simulink model "Microgrid_W"  (R2020a)
settings: Solver=ode15s  StartTime=0  StopTime=1440*1  MaxStep=1  RelTol=1e-3
libraries: simulink x4214, powerlib x685, simulink_extras x28, Microgrid_Library x18, powerlib_meascontrol x12
(part 39 of 48)

== system Microgrid_W/House 5 W1/Light 5/D5 ==
  Clock : Clock
  Constant : Constant
  Constant1 : Constant  Value=0
  Gain : Gain  Gain=t
  Interval Test : simulink/Logic and Bit Operations/Interval Test  IntervalClosedRight=on  uplimit=K_L4_Off_1+86400*4  IntervalClosedLeft=on  lowlimit=K_L4_On_1+86400*4  OutDataTypeStr=boolean
  Switch : Switch  Criteria=u2 > Threshold  Threshold=0.5
  Out1 : Outport  VectorParamsAs1DForOutWhenUnconnected=off
  wires:
  Clock/1 -> Gain/1
  Gain/1 -> Interval Test/1
  Constant/1 -> Switch/1
  Constant1/1 -> Switch/3
  Switch/1 -> Out1/1
  Interval Test/1 -> Switch/2

== system Microgrid_W/House 5 W1/Light 5/D6 ==
  Clock : Clock
  Constant : Constant
  Constant1 : Constant  Value=0
  Gain : Gain  Gain=t
  Interval Test : simulink/Logic and Bit Operations/Interval Test  IntervalClosedRight=on  uplimit=K_L4_Off_1+86400*5  IntervalClosedLeft=on  lowlimit=K_L4_On_1+86400*5  OutDataTypeStr=boolean
  Switch : Switch  Criteria=u2 > Threshold  Threshold=0.5
  Out1 : Outport  VectorParamsAs1DForOutWhenUnconnected=off
  wires:
  Clock/1 -> Gain/1
  Interval Test/1 -> Switch/2
  Switch/1 -> Out1/1
  Constant1/1 -> Switch/3
  Constant/1 -> Switch/1
  Gain/1 -> Interval Test/1

== system Microgrid_W/House 5 W1/Light 5/D7 ==
  Clock : Clock
  Constant : Constant
  Constant1 : Constant  Value=0
  Gain : Gain  Gain=t
  Interval Test : simulink/Logic and Bit Operations/Interval Test  IntervalClosedRight=on  uplimit=K_L4_Off_1+86400*6  IntervalClosedLeft=on  lowlimit=K_L4_On_1+86400*6  OutDataTypeStr=boolean
  Switch : Switch  Criteria=u2 > Threshold  Threshold=0.5
  Out1 : Outport  VectorParamsAs1DForOutWhenUnconnected=off
  wires:
  Clock/1 -> Gain/1
  Gain/1 -> Interval Test/1
  Constant/1 -> Switch/1
  Constant1/1 -> Switch/3
  Switch/1 -> Out1/1
  Interval Test/1 -> Switch/2

== system Microgrid_W/House 5 W1/Light 6/D1 ==
  Add : Sum
  Clock : Clock
  Constant : Constant
  Constant1 : Constant  Value=0
  Gain : Gain  Gain=t
  Interval Test : simulink/Logic and Bit Operations/Interval Test  IntervalClosedRight=on  uplimit=K_L5_Off_1  IntervalClosedLeft=on  lowlimit=K_L5_On_1  OutDataTypeStr=boolean
  Interval Test1 : simulink/Logic and Bit Operations/Interval Test  IntervalClosedRight=on  uplimit=K_L5_Off_2  IntervalClosedLeft=on  lowlimit=K_L5_On_2  OutDataTypeStr=boolean
  Switch : Switch  Criteria=u2 > Threshold  Threshold=0.5
  Switch1 : Switch  Criteria=u2 > Threshold  Threshold=0.5
  Out1 : Outport  VectorParamsAs1DForOutWhenUnconnected=off
  wires:
  Clock/1 -> Gain/1
  Interval Test/1 -> Switch/2
  Switch/1 -> Add/1
  Interval Test1/1 -> Switch1/2
  Add/1 -> Out1/1
  Constant1/1 -> Switch/3, Switch1/3
  Constant/1 -> Switch/1, Switch1/1
  Switch1/1 -> Add/2
  Gain/1 -> Interval Test1/1, Interval Test/1

== system Microgrid_W/House 5 W1/Light 6/D2 ==
  Add : Sum
  Clock : Clock
  Constant : Constant
  Constant1 : Constant  Value=0
  Gain : Gain  Gain=t
  Interval Test : simulink/Logic and Bit Operations/Interval Test  IntervalClosedRight=on  uplimit=K_L5_Off_1+86400  IntervalClosedLeft=on  lowlimit=K_L5_On_1+86400  OutDataTypeStr=boolean
  Interval Test1 : simulink/Logic and Bit Operations/Interval Test  IntervalClosedRight=on  uplimit=K_L5_Off_2+86400  IntervalClosedLeft=on  lowlimit=K_L5_On_2+86400  OutDataTypeStr=boolean
  Switch : Switch  Criteria=u2 > Threshold  Threshold=0.5
  Switch1 : Switch  Criteria=u2 > Threshold  Threshold=0.5
  Out1 : Outport  VectorParamsAs1DForOutWhenUnconnected=off
  wires:
  Clock/1 -> Gain/1
  Gain/1 -> Interval Test/1, Interval Test1/1
  Switch1/1 -> Add/2
  Constant/1 -> Switch1/1, Switch/1
  Constant1/1 -> Switch1/3, Switch/3
  Add/1 -> Out1/1
  Interval Test1/1 -> Switch1/2
  Switch/1 -> Add/1
  Interval Test/1 -> Switch/2

== system Microgrid_W/House 5 W1/Light 6/D3 ==
  Add : Sum
  Clock : Clock
  Constant : Constant
  Constant1 : Constant  Value=0
  Gain : Gain  Gain=t
  Interval Test : simulink/Logic and Bit Operations/Interval Test  IntervalClosedRight=on  uplimit=K_L5_Off_1+86400*2  IntervalClosedLeft=on  lowlimit=K_L5_On_1+86400*2  OutDataTypeStr=boolean
  Interval Test1 : simulink/Logic and Bit Operations/Interval Test  IntervalClosedRight=on  uplimit=K_L5_Off_2+86400*2  IntervalClosedLeft=on  lowlimit=K_L5_On_2+86400*2  OutDataTypeStr=boolean
  Switch : Switch  Criteria=u2 > Threshold  Threshold=0.5
  Switch1 : Switch  Criteria=u2 > Threshold  Threshold=0.5
  Out1 : Outport  VectorParamsAs1DForOutWhenUnconnected=off
  wires:
  Clock/1 -> Gain/1
  Interval Test/1 -> Switch/2
  Switch/1 -> Add/1
  Interval Test1/1 -> Switch1/2
  Add/1 -> Out1/1
  Constant1/1 -> Switch/3, Switch1/3
  Constant/1 -> Switch/1, Switch1/1
  Switch1/1 -> Add/2
  Gain/1 -> Interval Test1/1, Interval Test/1

== system Microgrid_W/House 5 W1/Light 6/D4 ==
  Add : Sum
  Clock : Clock
  Constant : Constant
  Constant1 : Constant  Value=0
  Gain : Gain  Gain=t
  Interval Test : simulink/Logic and Bit Operations/Interval Test  IntervalClosedRight=on  uplimit=K_L5_Off_1+86400*3  IntervalClosedLeft=on  lowlimit=K_L5_On_1+86400*3  OutDataTypeStr=boolean
  Interval Test1 : simulink/Logic and Bit Operations/Interval Test  IntervalClosedRight=on  uplimit=K_L5_Off_2+86400*3  IntervalClosedLeft=on  lowlimit=K_L5_On_2+86400*3  OutDataTypeStr=boolean
  Switch : Switch  Criteria=u2 > Threshold  Threshold=0.5
  Switch1 : Switch  Criteria=u2 > Threshold  Threshold=0.5
  Out1 : Outport  VectorParamsAs1DForOutWhenUnconnected=off
  wires:
  Clock/1 -> Gain/1
  Gain/1 -> Interval Test/1, Interval Test1/1
  Switch1/1 -> Add/2
  Constant/1 -> Switch1/1, Switch/1
  Constant1/1 -> Switch1/3, Switch/3
  Add/1 -> Out1/1
  Interval Test1/1 -> Switch1/2
  Switch/1 -> Add/1
  Interval Test/1 -> Switch/2

== system Microgrid_W/House 5 W1/Light 6/D5 ==
  Add : Sum
  Clock : Clock
  Constant : Constant
  Constant1 : Constant  Value=0
  Gain : Gain  Gain=t
  Interval Test : simulink/Logic and Bit Operations/Interval Test  IntervalClosedRight=on  uplimit=K_L5_Off_1+86400*4  IntervalClosedLeft=on  lowlimit=K_L5_On_1+86400*4  OutDataTypeStr=boolean
  Interval Test1 : simulink/Logic and Bit Operations/Interval Test  IntervalClosedRight=on  uplimit=K_L5_Off_2+86400*4  IntervalClosedLeft=on  lowlimit=K_L5_On_2+86400*4  OutDataTypeStr=boolean
  Switch : Switch  Criteria=u2 > Threshold  Threshold=0.5
  Switch1 : Switch  Criteria=u2 > Threshold  Threshold=0.5
  Out1 : Outport  VectorParamsAs1DForOutWhenUnconnected=off
  wires:
  Clock/1 -> Gain/1
  Interval Test/1 -> Switch/2
  Switch/1 -> Add/1
  Interval Test1/1 -> Switch1/2
  Add/1 -> Out1/1
  Constant1/1 -> Switch/3, Switch1/3
  Constant/1 -> Switch/1, Switch1/1
  Switch1/1 -> Add/2
  Gain/1 -> Interval Test1/1, Interval Test/1

== system Microgrid_W/House 5 W1/Light 6/D6 ==
  Add : Sum
  Clock : Clock
  Constant : Constant
  Constant1 : Constant  Value=0
  Gain : Gain  Gain=t
  Interval Test : simulink/Logic and Bit Operations/Interval Test  IntervalClosedRight=on  uplimit=K_L5_Off_1+86400*5  IntervalClosedLeft=on  lowlimit=K_L5_On_1+86400*5  OutDataTypeStr=boolean
  Interval Test1 : simulink/Logic and Bit Operations/Interval Test  IntervalClosedRight=on  uplimit=K_L5_Off_2+86400*5  IntervalClosedLeft=on  lowlimit=K_L5_On_2+86400*5  OutDataTypeStr=boolean
  Switch : Switch  Criteria=u2 > Threshold  Threshold=0.5
  Switch1 : Switch  Criteria=u2 > Threshold  Threshold=0.5
  Out1 : Outport  VectorParamsAs1DForOutWhenUnconnected=off
  wires:
  Clock/1 -> Gain/1
  Gain/1 -> Interval Test/1, Interval Test1/1
  Switch1/1 -> Add/2
  Constant/1 -> Switch1/1, Switch/1
  Constant1/1 -> Switch1/3, Switch/3
  Add/1 -> Out1/1
  Interval Test1/1 -> Switch1/2
  Switch/1 -> Add/1
  Interval Test/1 -> Switch/2

== system Microgrid_W/House 5 W1/Light 6/D7 ==
  Add : Sum
  Clock : Clock
  Constant : Constant
  Constant1 : Constant  Value=0
  Gain : Gain  Gain=t
  Interval Test : simulink/Logic and Bit Operations/Interval Test  IntervalClosedRight=on  uplimit=K_L5_Off_1+86400*6  IntervalClosedLeft=on  lowlimit=K_L5_On_1+86400*6  OutDataTypeStr=boolean
  Interval Test1 : simulink/Logic and Bit Operations/Interval Test  IntervalClosedRight=on  uplimit=K_L5_Off_2+86400*6  IntervalClosedLeft=on  lowlimit=K_L5_On_2+86400*6  OutDataTypeStr=boolean
  Switch : Switch  Criteria=u2 > Threshold  Threshold=0.5
  Switch1 : Switch  Criteria=u2 > Threshold  Threshold=0.5
  Out1 : Outport  VectorParamsAs1DForOutWhenUnconnected=off
  wires:
  Clock/1 -> Gain/1
  Interval Test/1 -> Switch/2
  Switch/1 -> Add/1
  Interval Test1/1 -> Switch1/2
  Add/1 -> Out1/1
  Constant1/1 -> Switch/3, Switch1/3
  Constant/1 -> Switch/1, Switch1/1
  Switch1/1 -> Add/2
  Gain/1 -> Interval Test1/1, Interval Test/1

== system Microgrid_W/House 5 W1/Light 7/D1 ==
  Clock : Clock
  Constant : Constant
  Constant1 : Constant  Value=0
  Gain : Gain  Gain=t
  Interval Test : simulink/Logic and Bit Operations/Interval Test  IntervalClosedRight=on  uplimit=K_L6_Off_1  IntervalClosedLeft=on  lowlimit=K_L6_On_1  OutDataTypeStr=boolean
  Switch : Switch  Criteria=u2 > Threshold  Threshold=0.5
  Out1 : Outport  VectorParamsAs1DForOutWhenUnconnected=off
  wires:
  Clock/1 -> Gain/1
  Gain/1 -> Interval Test/1
  Constant/1 -> Switch/1
  Constant1/1 -> Switch/3
  Switch/1 -> Out1/1
  Interval Test/1 -> Switch/2

== system Microgrid_W/House 5 W1/Light 7/D2 ==
  Clock : Clock
  Constant : Constant
  Constant1 : Constant  Value=0
  Gain : Gain  Gain=t
  Interval Test : simulink/Logic and Bit Operations/Interval Test  IntervalClosedRight=on  uplimit=K_L6_Off_1+86400  IntervalClosedLeft=on  lowlimit=K_L6_On_1+86400  OutDataTypeStr=boolean
  Switch : Switch  Criteria=u2 > Threshold  Threshold=0.5
  Out1 : Outport  VectorParamsAs1DForOutWhenUnconnected=off
  wires:
  Clock/1 -> Gain/1
  Interval Test/1 -> Switch/2
  Switch/1 -> Out1/1
  Constant1/1 -> Switch/3
  Constant/1 -> Switch/1
  Gain/1 -> Interval Test/1

== system Microgrid_W/House 5 W1/Light 7/D3 ==
  Clock : Clock
  Constant : Constant
  Constant1 : Constant  Value=0
  Gain : Gain  Gain=t
  Interval Test : simulink/Logic and Bit Operations/Interval Test  IntervalClosedRight=on  uplimit=K_L6_Off_1+86400*2  IntervalClosedLeft=on  lowlimit=K_L6_On_1+86400*2  OutDataTypeStr=boolean
  Switch : Switch  Criteria=u2 > Threshold  Threshold=0.5
  Out1 : Outport  VectorParamsAs1DForOutWhenUnconnected=off
  wires:
  Clock/1 -> Gain/1
  Gain/1 -> Interval Test/1
  Constant/1 -> Switch/1
  Constant1/1 -> Switch/3
  Switch/1 -> Out1/1
  Interval Test/1 -> Switch/2

== system Microgrid_W/House 5 W1/Light 7/D4 ==
  Clock : Clock
  Constant : Constant
  Constant1 : Constant  Value=0
  Gain : Gain  Gain=t
  Interval Test : simulink/Logic and Bit Operations/Interval Test  IntervalClosedRight=on  uplimit=K_L6_Off_1+86400*3  IntervalClosedLeft=on  lowlimit=K_L6_On_1+86400*3  OutDataTypeStr=boolean
  Switch : Switch  Criteria=u2 > Threshold  Threshold=0.5
  Out1 : Outport  VectorParamsAs1DForOutWhenUnconnected=off
  wires:
  Clock/1 -> Gain/1
  Interval Test/1 -> Switch/2
  Switch/1 -> Out1/1
  Constant1/1 -> Switch/3
  Constant/1 -> Switch/1
  Gain/1 -> Interval Test/1

== system Microgrid_W/House 5 W1/Light 7/D5 ==
  Clock : Clock
  Constant : Constant
  Constant1 : Constant  Value=0
  Gain : Gain  Gain=t
  Interval Test : simulink/Logic and Bit Operations/Interval Test  IntervalClosedRight=on  uplimit=K_L6_Off_1+86400*4  IntervalClosedLeft=on  lowlimit=K_L6_On_1+86400*4  OutDataTypeStr=boolean
  Switch : Switch  Criteria=u2 > Threshold  Threshold=0.5
  Out1 : Outport  VectorParamsAs1DForOutWhenUnconnected=off
  wires:
  Clock/1 -> Gain/1
  Gain/1 -> Interval Test/1
  Constant/1 -> Switch/1
  Constant1/1 -> Switch/3
  Switch/1 -> Out1/1
  Interval Test/1 -> Switch/2

== system Microgrid_W/House 5 W1/Light 7/D6 ==
  Clock : Clock
  Constant : Constant
  Constant1 : Constant  Value=0
  Gain : Gain  Gain=t
  Interval Test : simulink/Logic and Bit Operations/Interval Test  IntervalClosedRight=on  uplimit=K_L6_Off_1+86400*5  IntervalClosedLeft=on  lowlimit=K_L6_On_1+86400*5  OutDataTypeStr=boolean
  Switch : Switch  Criteria=u2 > Threshold  Threshold=0.5
  Out1 : Outport  VectorParamsAs1DForOutWhenUnconnected=off
  wires:
  Clock/1 -> Gain/1
  Interval Test/1 -> Switch/2
  Switch/1 -> Out1/1
  Constant1/1 -> Switch/3
  Constant/1 -> Switch/1
  Gain/1 -> Interval Test/1

== system Microgrid_W/House 5 W1/Light 7/D7 ==
  Clock : Clock
  Constant : Constant
  Constant1 : Constant  Value=0
  Gain : Gain  Gain=t
  Interval Test : simulink/Logic and Bit Operations/Interval Test  IntervalClosedRight=on  uplimit=K_L6_Off_1+86400*6  IntervalClosedLeft=on  lowlimit=K_L6_On_1+86400*6  OutDataTypeStr=boolean
  Switch : Switch  Criteria=u2 > Threshold  Threshold=0.5
  Out1 : Outport  VectorParamsAs1DForOutWhenUnconnected=off
  wires:
  Clock/1 -> Gain/1
  Gain/1 -> Interval Test/1
  Constant/1 -> Switch/1
  Constant1/1 -> Switch/3
  Switch/1 -> Out1/1
  Interval Test/1 -> Switch/2

== system Microgrid_W/House 5 W1/Oven/D1 ==
  Clock : Clock
  Constant : Constant
  Constant1 : Constant  Value=0
  Gain : Gain  Gain=t
  Interval Test : simulink/Logic and Bit Operations/Interval Test  IntervalClosedRight=on  uplimit=Oven_Off_1  IntervalClosedLeft=on  lowlimit=Oven_On_1  OutDataTypeStr=boolean
  Switch : Switch  Criteria=u2 > Threshold  Threshold=0.5
  Out1 : Outport  VectorParamsAs1DForOutWhenUnconnected=off
  wires:
  Clock/1 -> Gain/1
  Gain/1 -> Interval Test/1
  Constant/1 -> Switch/1
  Constant1/1 -> Switch/3
  Switch/1 -> Out1/1
  Interval Test/1 -> Switch/2

== system Microgrid_W/House 5 W1/Oven/D2 ==
  Clock : Clock
  Constant : Constant
  Constant1 : Constant  Value=0
  Gain : Gain  Gain=t
  Interval Test : simulink/Logic and Bit Operations/Interval Test  IntervalClosedRight=on  uplimit=Oven_Off_1+86400  IntervalClosedLeft=on  lowlimit=Oven_On_1+86400  OutDataTypeStr=boolean
  Switch : Switch  Criteria=u2 > Threshold  Threshold=0.5
  Out1 : Outport  VectorParamsAs1DForOutWhenUnconnected=off
  wires:
  Clock/1 -> Gain/1
  Interval Test/1 -> Switch/2
  Switch/1 -> Out1/1
  Constant1/1 -> Switch/3
  Constant/1 -> Switch/1
  Gain/1 -> Interval Test/1

== system Microgrid_W/House 5 W1/Oven/D3 ==
  Clock : Clock
  Constant : Constant
  Constant1 : Constant  Value=0
  Gain : Gain  Gain=t
  Interval Test : simulink/Logic and Bit Operations/Interval Test  IntervalClosedRight=on  uplimit=Oven_Off_1+86400*2  IntervalClosedLeft=on  lowlimit=Oven_On_1+86400*2  OutDataTypeStr=boolean
  Switch : Switch  Criteria=u2 > Threshold  Threshold=0.5
  Out1 : Outport  VectorParamsAs1DForOutWhenUnconnected=off
  wires:
  Clock/1 -> Gain/1
  Gain/1 -> Interval Test/1
  Constant/1 -> Switch/1
  Constant1/1 -> Switch/3
  Switch/1 -> Out1/1
  Interval Test/1 -> Switch/2

== system Microgrid_W/House 5 W1/Oven/D4 ==
  Clock : Clock
  Constant : Constant
  Constant1 : Constant  Value=0
  Gain : Gain  Gain=t
  Interval Test : simulink/Logic and Bit Operations/Interval Test  IntervalClosedRight=on  uplimit=Oven_Off_1+86400*3  IntervalClosedLeft=on  lowlimit=Oven_On_1+86400*3  OutDataTypeStr=boolean
  Switch : Switch  Criteria=u2 > Threshold  Threshold=0.5
  Out1 : Outport  VectorParamsAs1DForOutWhenUnconnected=off
  wires:
  Clock/1 -> Gain/1
  Interval Test/1 -> Switch/2
  Switch/1 -> Out1/1
  Constant1/1 -> Switch/3
  Constant/1 -> Switch/1
  Gain/1 -> Interval Test/1

== system Microgrid_W/House 5 W1/Oven/D5 ==
  Clock : Clock
  Constant : Constant
  Constant1 : Constant  Value=0
  Gain : Gain  Gain=t
  Interval Test : simulink/Logic and Bit Operations/Interval Test  IntervalClosedRight=on  uplimit=Oven_Off_1+86400*4  IntervalClosedLeft=on  lowlimit=Oven_On_1+86400*4  OutDataTypeStr=boolean
  Switch : Switch  Criteria=u2 > Threshold  Threshold=0.5
  Out1 : Outport  VectorParamsAs1DForOutWhenUnconnected=off
  wires:
  Clock/1 -> Gain/1
  Gain/1 -> Interval Test/1
  Constant/1 -> Switch/1
  Constant1/1 -> Switch/3
  Switch/1 -> Out1/1
  Interval Test/1 -> Switch/2

== system Microgrid_W/House 5 W1/Oven/D6 ==
  Clock : Clock
  Constant : Constant
  Constant1 : Constant  Value=0
  Gain : Gain  Gain=t
  Interval Test : simulink/Logic and Bit Operations/Interval Test  IntervalClosedRight=on  uplimit=Oven_Off_1+86400*5  IntervalClosedLeft=on  lowlimit=Oven_On_1+86400*5  OutDataTypeStr=boolean
  Switch : Switch  Criteria=u2 > Threshold  Threshold=0.5
  Out1 : Outport  VectorParamsAs1DForOutWhenUnconnected=off
  wires:
  Clock/1 -> Gain/1
  Interval Test/1 -> Switch/2
  Switch/1 -> Out1/1
  Constant1/1 -> Switch/3
  Constant/1 -> Switch/1
  Gain/1 -> Interval Test/1

== system Microgrid_W/House 5 W1/Oven/D7 ==
  Clock : Clock
  Constant : Constant
  Constant1 : Constant  Value=0
  Gain : Gain  Gain=t
  Interval Test : simulink/Logic and Bit Operations/Interval Test  IntervalClosedRight=on  uplimit=Oven_Off_1+86400*6  IntervalClosedLeft=on  lowlimit=Oven_On_1+86400*6  OutDataTypeStr=boolean
  Switch : Switch  Criteria=u2 > Threshold  Threshold=0.5
  Out1 : Outport  VectorParamsAs1DForOutWhenUnconnected=off
  wires:
  Clock/1 -> Gain/1
  Gain/1 -> Interval Test/1
  Constant/1 -> Switch/1
  Constant1/1 -> Switch/3
  Switch/1 -> Out1/1
  Interval Test/1 -> Switch/2

== system Microgrid_W/House 5 W1/Phone_Charger/D1 ==
  Add : Sum
  Clock : Clock
  Constant : Constant
  Constant1 : Constant  Value=0
  Gain : Gain  Gain=t
  Interval Test : simulink/Logic and Bit Operations/Interval Test  IntervalClosedRight=on  uplimit=Phone_C_1_Off_a  IntervalClosedLeft=on  lowlimit=Phone_C_1_On_a  OutDataTypeStr=boolean
  Interval Test1 : simulink/Logic and Bit Operations/Interval Test  IntervalClosedRight=on  uplimit=Phone_C_1_Off_b  IntervalClosedLeft=on  lowlimit=Phone_C_1_On_b  OutDataTypeStr=boolean
  Switch : Switch  Criteria=u2 > Threshold  Threshold=0.5
  Switch1 : Switch  Criteria=u2 > Threshold  Threshold=0.5
  Out1 : Outport  VectorParamsAs1DForOutWhenUnconnected=off
  wires:
  Clock/1 -> Gain/1
  Interval Test/1 -> Switch/2
  Switch/1 -> Add/1
  Interval Test1/1 -> Switch1/2
  Add/1 -> Out1/1
  Constant1/1 -> Switch/3, Switch1/3
  Constant/1 -> Switch/1, Switch1/1
  Switch1/1 -> Add/2
  Gain/1 -> Interval Test1/1, Interval Test/1

== system Microgrid_W/House 5 W1/Phone_Charger/D10 ==
  Add : Sum
  Clock : Clock
  Constant : Constant
  Constant1 : Constant  Value=0
  Gain : Gain  Gain=t
  Interval Test : simulink/Logic and Bit Operations/Interval Test  IntervalClosedRight=on  uplimit=Phone_C_2_Off_a+86400*2  IntervalClosedLeft=on  lowlimit=Phone_C_2_On_a+86400*2  OutDataTypeStr=boolean
  Interval Test1 : simulink/Logic and Bit Operations/Interval Test  IntervalClosedRight=on  uplimit=Phone_C_2_Off_b+86400*2  IntervalClosedLeft=on  lowlimit=Phone_C_2_On_b+86400*2  OutDataTypeStr=boolean
  Switch : Switch  Criteria=u2 > Threshold  Threshold=0.5
  Switch1 : Switch  Criteria=u2 > Threshold  Threshold=0.5
  Out1 : Outport  VectorParamsAs1DForOutWhenUnconnected=off
  wires:
  Clock/1 -> Gain/1
  Gain/1 -> Interval Test/1, Interval Test1/1
  Switch1/1 -> Add/2
  Constant/1 -> Switch1/1, Switch/1
  Constant1/1 -> Switch1/3, Switch/3
  Add/1 -> Out1/1
  Interval Test1/1 -> Switch1/2
  Switch/1 -> Add/1
  Interval Test/1 -> Switch/2

== system Microgrid_W/House 5 W1/Phone_Charger/D11 ==
  Add : Sum
  Clock : Clock
  Constant : Constant
  Constant1 : Constant  Value=0
  Gain : Gain  Gain=t
  Interval Test : simulink/Logic and Bit Operations/Interval Test  IntervalClosedRight=on  uplimit=Phone_C_2_Off_a+86400*3  IntervalClosedLeft=on  lowlimit=Phone_C_2_On_a+86400*3  OutDataTypeStr=boolean
  Interval Test1 : simulink/Logic and Bit Operations/Interval Test  IntervalClosedRight=on  uplimit=Phone_C_2_Off_b+86400*3  IntervalClosedLeft=on  lowlimit=Phone_C_2_On_b+86400*3  OutDataTypeStr=boolean
  Switch : Switch  Criteria=u2 > Threshold  Threshold=0.5
  Switch1 : Switch  Criteria=u2 > Threshold  Threshold=0.5
  Out1 : Outport  VectorParamsAs1DForOutWhenUnconnected=off
  wires:
  Clock/1 -> Gain/1
  Interval Test/1 -> Switch/2
  Switch/1 -> Add/1
  Interval Test1/1 -> Switch1/2
  Add/1 -> Out1/1
  Constant1/1 -> Switch/3, Switch1/3
  Constant/1 -> Switch/1, Switch1/1
  Switch1/1 -> Add/2
  Gain/1 -> Interval Test1/1, Interval Test/1

== system Microgrid_W/House 5 W1/Phone_Charger/D12 ==
  Add : Sum
  Clock : Clock
  Constant : Constant
  Constant1 : Constant  Value=0
  Gain : Gain  Gain=t
  Interval Test : simulink/Logic and Bit Operations/Interval Test  IntervalClosedRight=on  uplimit=Phone_C_2_Off_a+86400*4  IntervalClosedLeft=on  lowlimit=Phone_C_2_On_a+86400*4  OutDataTypeStr=boolean
  Interval Test1 : simulink/Logic and Bit Operations/Interval Test  IntervalClosedRight=on  uplimit=Phone_C_2_Off_b+86400*4  IntervalClosedLeft=on  lowlimit=Phone_C_2_On_b+86400*4  OutDataTypeStr=boolean
  Switch : Switch  Criteria=u2 > Threshold  Threshold=0.5
  Switch1 : Switch  Criteria=u2 > Threshold  Threshold=0.5
  Out1 : Outport  VectorParamsAs1DForOutWhenUnconnected=off
  wires:
  Clock/1 -> Gain/1
  Gain/1 -> Interval Test/1, Interval Test1/1
  Switch1/1 -> Add/2
  Constant/1 -> Switch1/1, Switch/1
  Constant1/1 -> Switch1/3, Switch/3
  Add/1 -> Out1/1
  Interval Test1/1 -> Switch1/2
  Switch/1 -> Add/1
  Interval Test/1 -> Switch/2

== system Microgrid_W/House 5 W1/Phone_Charger/D13 ==
  Add : Sum
  Clock : Clock
  Constant : Constant
  Constant1 : Constant  Value=0
  Gain : Gain  Gain=t
  Interval Test : simulink/Logic and Bit Operations/Interval Test  IntervalClosedRight=on  uplimit=Phone_C_2_Off_a+86400*5  IntervalClosedLeft=on  lowlimit=Phone_C_2_On_a+86400*5  OutDataTypeStr=boolean
  Interval Test1 : simulink/Logic and Bit Operations/Interval Test  IntervalClosedRight=on  uplimit=Phone_C_2_Off_b+86400*5  IntervalClosedLeft=on  lowlimit=Phone_C_2_On_b+86400*5  OutDataTypeStr=boolean
  Switch : Switch  Criteria=u2 > Threshold  Threshold=0.5
  Switch1 : Switch  Criteria=u2 > Threshold  Threshold=0.5
  Out1 : Outport  VectorParamsAs1DForOutWhenUnconnected=off
  wires:
  Clock/1 -> Gain/1
  Interval Test/1 -> Switch/2
  Switch/1 -> Add/1
  Interval Test1/1 -> Switch1/2
  Add/1 -> Out1/1
  Constant1/1 -> Switch/3, Switch1/3
  Constant/1 -> Switch/1, Switch1/1
  Switch1/1 -> Add/2
  Gain/1 -> Interval Test1/1, Interval Test/1

== system Microgrid_W/House 5 W1/Phone_Charger/D14 ==
  Add : Sum
  Clock : Clock
  Constant : Constant
  Constant1 : Constant  Value=0
  Gain : Gain  Gain=t
  Interval Test : simulink/Logic and Bit Operations/Interval Test  IntervalClosedRight=on  uplimit=Phone_C_2_Off_a+86400*6  IntervalClosedLeft=on  lowlimit=Phone_C_2_On_a+86400*6  OutDataTypeStr=boolean
  Interval Test1 : simulink/Logic and Bit Operations/Interval Test  IntervalClosedRight=on  uplimit=Phone_C_2_Off_b+86400*6  IntervalClosedLeft=on  lowlimit=Phone_C_2_On_b+86400*6  OutDataTypeStr=boolean
  Switch : Switch  Criteria=u2 > Threshold  Threshold=0.5
  Switch1 : Switch  Criteria=u2 > Threshold  Threshold=0.5
  Out1 : Outport  VectorParamsAs1DForOutWhenUnconnected=off
  wires:
  Clock/1 -> Gain/1
  Gain/1 -> Interval Test/1, Interval Test1/1
  Switch1/1 -> Add/2
  Constant/1 -> Switch1/1, Switch/1
  Constant1/1 -> Switch1/3, Switch/3
  Add/1 -> Out1/1
  Interval Test1/1 -> Switch1/2
  Switch/1 -> Add/1
  Interval Test/1 -> Switch/2

== system Microgrid_W/House 5 W1/Phone_Charger/D15 ==
  Add : Sum
  Clock : Clock
  Constant : Constant
  Constant1 : Constant  Value=0
  Gain : Gain  Gain=t
  Interval Test : simulink/Logic and Bit Operations/Interval Test  IntervalClosedRight=on  uplimit=Phone_C_3_Off_a+86400  IntervalClosedLeft=on  lowlimit=Phone_C_3_On_a+86400  OutDataTypeStr=boolean
  Interval Test1 : simulink/Logic and Bit Operations/Interval Test  IntervalClosedRight=on  uplimit=Phone_C_3_Off_b+86400  IntervalClosedLeft=on  lowlimit=Phone_C_3_On_b+86400  OutDataTypeStr=boolean
  Switch : Switch  Criteria=u2 > Threshold  Threshold=0.5
  Switch1 : Switch  Criteria=u2 > Threshold  Threshold=0.5
  Out1 : Outport  VectorParamsAs1DForOutWhenUnconnected=off
  wires:
  Clock/1 -> Gain/1
  Gain/1 -> Interval Test/1, Interval Test1/1
  Switch1/1 -> Add/2
  Constant/1 -> Switch1/1, Switch/1
  Constant1/1 -> Switch1/3, Switch/3
  Add/1 -> Out1/1
  Interval Test1/1 -> Switch1/2
  Switch/1 -> Add/1
  Interval Test/1 -> Switch/2

== system Microgrid_W/House 5 W1/Phone_Charger/D16 ==
  Add : Sum
  Clock : Clock
  Constant : Constant
  Constant1 : Constant  Value=0
  Gain : Gain  Gain=t
  Interval Test : simulink/Logic and Bit Operations/Interval Test  IntervalClosedRight=on  uplimit=Phone_C_3_Off_a+86400*2  IntervalClosedLeft=on  lowlimit=Phone_C_3_On_a+86400*2  OutDataTypeStr=boolean
  Interval Test1 : simulink/Logic and Bit Operations/Interval Test  IntervalClosedRight=on  uplimit=Phone_C_3_Off_b+86400*2  IntervalClosedLeft=on  lowlimit=Phone_C_3_On_b+86400*2  OutDataTypeStr=boolean
  Switch : Switch  Criteria=u2 > Threshold  Threshold=0.5
  Switch1 : Switch  Criteria=u2 > Threshold  Threshold=0.5
  Out1 : Outport  VectorParamsAs1DForOutWhenUnconnected=off
  wires:
  Clock/1 -> Gain/1
  Interval Test/1 -> Switch/2
  Switch/1 -> Add/1
  Interval Test1/1 -> Switch1/2
  Add/1 -> Out1/1
  Constant1/1 -> Switch/3, Switch1/3
  Constant/1 -> Switch/1, Switch1/1
  Switch1/1 -> Add/2
  Gain/1 -> Interval Test1/1, Interval Test/1

== system Microgrid_W/House 5 W1/Phone_Charger/D17 ==
  Add : Sum
  Clock : Clock
  Constant : Constant
  Constant1 : Constant  Value=0
  Gain : Gain  Gain=t
  Interval Test : simulink/Logic and Bit Operations/Interval Test  IntervalClosedRight=on  uplimit=Phone_C_3_Off_a+86400*3  IntervalClosedLeft=on  lowlimit=Phone_C_3_On_a+86400*3  OutDataTypeStr=boolean
  Interval Test1 : simulink/Logic and Bit Operations/Interval Test  IntervalClosedRight=on  uplimit=Phone_C_3_Off_b+86400*3  IntervalClosedLeft=on  lowlimit=Phone_C_3_On_b+86400*3  OutDataTypeStr=boolean
  Switch : Switch  Criteria=u2 > Threshold  Threshold=0.5
  Switch1 : Switch  Criteria=u2 > Threshold  Threshold=0.5
  Out1 : Outport  VectorParamsAs1DForOutWhenUnconnected=off
  wires:
  Clock/1 -> Gain/1
  Gain/1 -> Interval Test/1, Interval Test1/1
  Switch1/1 -> Add/2
  Constant/1 -> Switch1/1, Switch/1
  Constant1/1 -> Switch1/3, Switch/3
  Add/1 -> Out1/1
  Interval Test1/1 -> Switch1/2
  Switch/1 -> Add/1
  Interval Test/1 -> Switch/2

== system Microgrid_W/House 5 W1/Phone_Charger/D18 ==
  Add : Sum
  Clock : Clock
  Constant : Constant
  Constant1 : Constant  Value=0
  Gain : Gain  Gain=t
  Interval Test : simulink/Logic and Bit Operations/Interval Test  IntervalClosedRight=on  uplimit=Phone_C_3_Off_a+86400*4  IntervalClosedLeft=on  lowlimit=Phone_C_3_On_a+86400*4  OutDataTypeStr=boolean
  Interval Test1 : simulink/Logic and Bit Operations/Interval Test  IntervalClosedRight=on  uplimit=Phone_C_3_Off_b+86400*4  IntervalClosedLeft=on  lowlimit=Phone_C_3_On_b+86400*4  OutDataTypeStr=boolean
  Switch : Switch  Criteria=u2 > Threshold  Threshold=0.5
  Switch1 : Switch  Criteria=u2 > Threshold  Threshold=0.5
  Out1 : Outport  VectorParamsAs1DForOutWhenUnconnected=off
  wires:
  Clock/1 -> Gain/1
  Interval Test/1 -> Switch/2
  Switch/1 -> Add/1
  Interval Test1/1 -> Switch1/2
  Add/1 -> Out1/1
  Constant1/1 -> Switch/3, Switch1/3
  Constant/1 -> Switch/1, Switch1/1
  Switch1/1 -> Add/2
  Gain/1 -> Interval Test1/1, Interval Test/1

== system Microgrid_W/House 5 W1/Phone_Charger/D19 ==
  Add : Sum
  Clock : Clock
  Constant : Constant
  Constant1 : Constant  Value=0
  Gain : Gain  Gain=t
  Interval Test : simulink/Logic and Bit Operations/Interval Test  IntervalClosedRight=on  uplimit=Phone_C_3_Off_a+86400*5  IntervalClosedLeft=on  lowlimit=Phone_C_3_On_a+86400*5  OutDataTypeStr=boolean
  Interval Test1 : simulink/Logic and Bit Operations/Interval Test  IntervalClosedRight=on  uplimit=Phone_C_3_Off_b+86400*5  IntervalClosedLeft=on  lowlimit=Phone_C_3_On_b+86400*5  OutDataTypeStr=boolean
  Switch : Switch  Criteria=u2 > Threshold  Threshold=0.5
  Switch1 : Switch  Criteria=u2 > Threshold  Threshold=0.5
  Out1 : Outport  VectorParamsAs1DForOutWhenUnconnected=off
  wires:
  Clock/1 -> Gain/1
  Gain/1 -> Interval Test/1, Interval Test1/1
  Switch1/1 -> Add/2
  Constant/1 -> Switch1/1, Switch/1
  Constant1/1 -> Switch1/3, Switch/3
  Add/1 -> Out1/1
  Interval Test1/1 -> Switch1/2
  Switch/1 -> Add/1
  Interval Test/1 -> Switch/2

== system Microgrid_W/House 5 W1/Phone_Charger/D2 ==
  Add : Sum
  Clock : Clock
  Constant : Constant
  Constant1 : Constant  Value=0
  Gain : Gain  Gain=t
  Interval Test : simulink/Logic and Bit Operations/Interval Test  IntervalClosedRight=on  uplimit=Phone_C_1_Off_a+86400  IntervalClosedLeft=on  lowlimit=Phone_C_1_On_a+86400  OutDataTypeStr=boolean
  Interval Test1 : simulink/Logic and Bit Operations/Interval Test  IntervalClosedRight=on  uplimit=Phone_C_1_Off_b+86400  IntervalClosedLeft=on  lowlimit=Phone_C_1_On_b+86400  OutDataTypeStr=boolean
  Switch : Switch  Criteria=u2 > Threshold  Threshold=0.5
  Switch1 : Switch  Criteria=u2 > Threshold  Threshold=0.5
  Out1 : Outport  VectorParamsAs1DForOutWhenUnconnected=off
  wires:
  Clock/1 -> Gain/1
  Gain/1 -> Interval Test/1, Interval Test1/1
  Switch1/1 -> Add/2
  Constant/1 -> Switch1/1, Switch/1
  Constant1/1 -> Switch1/3, Switch/3
  Add/1 -> Out1/1
  Interval Test1/1 -> Switch1/2
  Switch/1 -> Add/1
  Interval Test/1 -> Switch/2

== system Microgrid_W/House 5 W1/Phone_Charger/D20 ==
  Add : Sum
  Clock : Clock
  Constant : Constant
  Constant1 : Constant  Value=0
  Gain : Gain  Gain=t
  Interval Test : simulink/Logic and Bit Operations/Interval Test  IntervalClosedRight=on  uplimit=Phone_C_3_Off_a  IntervalClosedLeft=on  lowlimit=Phone_C_3_On_a  OutDataTypeStr=boolean
  Interval Test1 : simulink/Logic and Bit Operations/Interval Test  IntervalClosedRight=on  uplimit=Phone_C_3_Off_b  IntervalClosedLeft=on  lowlimit=Phone_C_3_On_b  OutDataTypeStr=boolean
  Switch : Switch  Criteria=u2 > Threshold  Threshold=0.5
  Switch1 : Switch  Criteria=u2 > Threshold  Threshold=0.5
  Out1 : Outport  VectorParamsAs1DForOutWhenUnconnected=off
  wires:
  Clock/1 -> Gain/1
  Interval Test/1 -> Switch/2
  Switch/1 -> Add/1
  Interval Test1/1 -> Switch1/2
  Add/1 -> Out1/1
  Constant1/1 -> Switch/3, Switch1/3
  Constant/1 -> Switch/1, Switch1/1
  Switch1/1 -> Add/2
  Gain/1 -> Interval Test1/1, Interval Test/1

== system Microgrid_W/House 5 W1/Phone_Charger/D21 ==
  Add : Sum
  Clock : Clock
  Constant : Constant
  Constant1 : Constant  Value=0
  Gain : Gain  Gain=t
  Interval Test : simulink/Logic and Bit Operations/Interval Test  IntervalClosedRight=on  uplimit=Phone_C_3_Off_a+86400*6  IntervalClosedLeft=on  lowlimit=Phone_C_3_On_a+86400*6  OutDataTypeStr=boolean
  Interval Test1 : simulink/Logic and Bit Operations/Interval Test  IntervalClosedRight=on  uplimit=Phone_C_3_Off_b+86400*6  IntervalClosedLeft=on  lowlimit=Phone_C_3_On_b+86400*6  OutDataTypeStr=boolean
  Switch : Switch  Criteria=u2 > Threshold  Threshold=0.5
  Switch1 : Switch  Criteria=u2 > Threshold  Threshold=0.5
  Out1 : Outport  VectorParamsAs1DForOutWhenUnconnected=off
  wires:
  Clock/1 -> Gain/1
  Interval Test/1 -> Switch/2
  Switch/1 -> Add/1
  Interval Test1/1 -> Switch1/2
  Add/1 -> Out1/1
  Constant1/1 -> Switch/3, Switch1/3
  Constant/1 -> Switch/1, Switch1/1
  Switch1/1 -> Add/2
  Gain/1 -> Interval Test1/1, Interval Test/1

== system Microgrid_W/House 5 W1/Phone_Charger/D3 ==
  Add : Sum
  Clock : Clock
  Constant : Constant
  Constant1 : Constant  Value=0
  Gain : Gain  Gain=t
  Interval Test : simulink/Logic and Bit Operations/Interval Test  IntervalClosedRight=on  uplimit=Phone_C_1_Off_a+86400*2  IntervalClosedLeft=on  lowlimit=Phone_C_1_On_a+86400*2  OutDataTypeStr=boolean
  Interval Test1 : simulink/Logic and Bit Operations/Interval Test  IntervalClosedRight=on  uplimit=Phone_C_1_Off_b+86400*2  IntervalClosedLeft=on  lowlimit=Phone_C_1_On_b+86400*2  OutDataTypeStr=boolean
  Switch : Switch  Criteria=u2 > Threshold  Threshold=0.5
  Switch1 : Switch  Criteria=u2 > Threshold  Threshold=0.5
  Out1 : Outport  VectorParamsAs1DForOutWhenUnconnected=off
  wires:
  Clock/1 -> Gain/1
  Interval Test/1 -> Switch/2
  Switch/1 -> Add/1
  Interval Test1/1 -> Switch1/2
  Add/1 -> Out1/1
  Constant1/1 -> Switch/3, Switch1/3
  Constant/1 -> Switch/1, Switch1/1
  Switch1/1 -> Add/2
  Gain/1 -> Interval Test1/1, Interval Test/1

== system Microgrid_W/House 5 W1/Phone_Charger/D4 ==
  Add : Sum
  Clock : Clock
  Constant : Constant
  Constant1 : Constant  Value=0
  Gain : Gain  Gain=t
  Interval Test : simulink/Logic and Bit Operations/Interval Test  IntervalClosedRight=on  uplimit=Phone_C_1_Off_a+86400*3  IntervalClosedLeft=on  lowlimit=Phone_C_1_On_a+86400*3  OutDataTypeStr=boolean
  Interval Test1 : simulink/Logic and Bit Operations/Interval Test  IntervalClosedRight=on  uplimit=Phone_C_1_Off_b+86400*3  IntervalClosedLeft=on  lowlimit=Phone_C_1_On_b+86400*3  OutDataTypeStr=boolean
  Switch : Switch  Criteria=u2 > Threshold  Threshold=0.5
  Switch1 : Switch  Criteria=u2 > Threshold  Threshold=0.5
  Out1 : Outport  VectorParamsAs1DForOutWhenUnconnected=off
  wires:
  Clock/1 -> Gain/1
  Gain/1 -> Interval Test/1, Interval Test1/1
  Switch1/1 -> Add/2
  Constant/1 -> Switch1/1, Switch/1
  Constant1/1 -> Switch1/3, Switch/3
  Add/1 -> Out1/1
  Interval Test1/1 -> Switch1/2
  Switch/1 -> Add/1
  Interval Test/1 -> Switch/2

== system Microgrid_W/House 5 W1/Phone_Charger/D5 ==
  Add : Sum
  Clock : Clock
  Constant : Constant
  Constant1 : Constant  Value=0
  Gain : Gain  Gain=t
  Interval Test : simulink/Logic and Bit Operations/Interval Test  IntervalClosedRight=on  uplimit=Phone_C_1_Off_a+86400*4  IntervalClosedLeft=on  lowlimit=Phone_C_1_On_a+86400*4  OutDataTypeStr=boolean
  Interval Test1 : simulink/Logic and Bit Operations/Interval Test  IntervalClosedRight=on  uplimit=Phone_C_1_Off_b+86400*4  IntervalClosedLeft=on  lowlimit=Phone_C_1_On_b+86400*4  OutDataTypeStr=boolean
  Switch : Switch  Criteria=u2 > Threshold  Threshold=0.5
  Switch1 : Switch  Criteria=u2 > Threshold  Threshold=0.5
  Out1 : Outport  VectorParamsAs1DForOutWhenUnconnected=off
  wires:
  Clock/1 -> Gain/1
  Interval Test/1 -> Switch/2
  Switch/1 -> Add/1
  Interval Test1/1 -> Switch1/2
  Add/1 -> Out1/1
  Constant1/1 -> Switch/3, Switch1/3
  Constant/1 -> Switch/1, Switch1/1
  Switch1/1 -> Add/2
  Gain/1 -> Interval Test1/1, Interval Test/1

== system Microgrid_W/House 5 W1/Phone_Charger/D6 ==
  Add : Sum
  Clock : Clock
  Constant : Constant
  Constant1 : Constant  Value=0
  Gain : Gain  Gain=t
  Interval Test : simulink/Logic and Bit Operations/Interval Test  IntervalClosedRight=on  uplimit=Phone_C_1_Off_a+86400*5  IntervalClosedLeft=on  lowlimit=Phone_C_1_On_a+86400*5  OutDataTypeStr=boolean
  Interval Test1 : simulink/Logic and Bit Operations/Interval Test  IntervalClosedRight=on  uplimit=Phone_C_1_Off_b+86400*5  IntervalClosedLeft=on  lowlimit=Phone_C_1_On_b+86400*5  OutDataTypeStr=boolean
  Switch : Switch  Criteria=u2 > Threshold  Threshold=0.5
  Switch1 : Switch  Criteria=u2 > Threshold  Threshold=0.5
  Out1 : Outport  VectorParamsAs1DForOutWhenUnconnected=off
  wires:
  Clock/1 -> Gain/1
  Gain/1 -> Interval Test/1, Interval Test1/1
  Switch1/1 -> Add/2
  Constant/1 -> Switch1/1, Switch/1
  Constant1/1 -> Switch1/3, Switch/3
  Add/1 -> Out1/1
  Interval Test1/1 -> Switch1/2
  Switch/1 -> Add/1
  Interval Test/1 -> Switch/2

== system Microgrid_W/House 5 W1/Phone_Charger/D7 ==
  Add : Sum
  Clock : Clock
  Constant : Constant
  Constant1 : Constant  Value=0
  Gain : Gain  Gain=t
  Interval Test : simulink/Logic and Bit Operations/Interval Test  IntervalClosedRight=on  uplimit=Phone_C_1_Off_a+86400*6  IntervalClosedLeft=on  lowlimit=Phone_C_1_On_a+86400*6  OutDataTypeStr=boolean
  Interval Test1 : simulink/Logic and Bit Operations/Interval Test  IntervalClosedRight=on  uplimit=Phone_C_1_Off_b+86400*6  IntervalClosedLeft=on  lowlimit=Phone_C_1_On_b+86400*6  OutDataTypeStr=boolean
  Switch : Switch  Criteria=u2 > Threshold  Threshold=0.5
  Switch1 : Switch  Criteria=u2 > Threshold  Threshold=0.5
  Out1 : Outport  VectorParamsAs1DForOutWhenUnconnected=off
  wires:
  Clock/1 -> Gain/1
  Interval Test/1 -> Switch/2
  Switch/1 -> Add/1
  Interval Test1/1 -> Switch1/2
  Add/1 -> Out1/1
  Constant1/1 -> Switch/3, Switch1/3
  Constant/1 -> Switch/1, Switch1/1
  Switch1/1 -> Add/2
  Gain/1 -> Interval Test1/1, Interval Test/1

== system Microgrid_W/House 5 W1/Phone_Charger/D8 ==
  Add : Sum
  Clock : Clock
  Constant : Constant
  Constant1 : Constant  Value=0
  Gain : Gain  Gain=t
  Interval Test : simulink/Logic and Bit Operations/Interval Test  IntervalClosedRight=on  uplimit=Phone_C_2_Off_a  IntervalClosedLeft=on  lowlimit=Phone_C_2_On_a  OutDataTypeStr=boolean
  Interval Test1 : simulink/Logic and Bit Operations/Interval Test  IntervalClosedRight=on  uplimit=Phone_C_2_Off_b  IntervalClosedLeft=on  lowlimit=Phone_C_2_On_b  OutDataTypeStr=boolean
  Switch : Switch  Criteria=u2 > Threshold  Threshold=0.5
  Switch1 : Switch  Criteria=u2 > Threshold  Threshold=0.5
  Out1 : Outport  VectorParamsAs1DForOutWhenUnconnected=off
  wires:
  Clock/1 -> Gain/1
  Gain/1 -> Interval Test/1, Interval Test1/1
  Switch1/1 -> Add/2
  Constant/1 -> Switch1/1, Switch/1
  Constant1/1 -> Switch1/3, Switch/3
  Add/1 -> Out1/1
  Interval Test1/1 -> Switch1/2
  Switch/1 -> Add/1
  Interval Test/1 -> Switch/2

== system Microgrid_W/House 5 W1/Phone_Charger/D9 ==
  Add : Sum
  Clock : Clock
  Constant : Constant
  Constant1 : Constant  Value=0
  Gain : Gain  Gain=t
  Interval Test : simulink/Logic and Bit Operations/Interval Test  IntervalClosedRight=on  uplimit=Phone_C_2_Off_a+86400  IntervalClosedLeft=on  lowlimit=Phone_C_2_On_a+86400  OutDataTypeStr=boolean
  Interval Test1 : simulink/Logic and Bit Operations/Interval Test  IntervalClosedRight=on  uplimit=Phone_C_2_Off_b+86400  IntervalClosedLeft=on  lowlimit=Phone_C_2_On_b+86400  OutDataTypeStr=boolean
  Switch : Switch  Criteria=u2 > Threshold  Threshold=0.5
  Switch1 : Switch  Criteria=u2 > Threshold  Threshold=0.5
  Out1 : Outport  VectorParamsAs1DForOutWhenUnconnected=off
  wires:
  Clock/1 -> Gain/1
  Interval Test/1 -> Switch/2
  Switch/1 -> Add/1
  Interval Test1/1 -> Switch1/2
  Add/1 -> Out1/1
  Constant1/1 -> Switch/3, Switch1/3
  Constant/1 -> Switch/1, Switch1/1
  Switch1/1 -> Add/2
  Gain/1 -> Interval Test1/1, Interval Test/1

== system Microgrid_W/House 5 W1/Refrigerator/Subsystem ==
  In1 : Inport
  Add : Sum
  Cc : Constant  Value=2.7
  Constant : Constant  Value=150
  Divide{,1..3} (4 alike) : Product  Inputs=*/
  Gain : Gain  Gain=1/(60)
  Integrator : Integrator
  Off : Constant  Value=0
  Product{,1..3} (4 alike) : Product
  Rec : Constant  Value=0.35
  Rec1 : Constant
  Ri : Constant  Value=2
  Scope : Scope
  Subtract : Sum  Inputs=++-
  Switch : Switch  Criteria=u2 > Threshold  Threshold=0.5
  Switch1 : Switch  Criteria=u2 > Threshold  Threshold=0.5
  T_I : Constant  Value=T_Initial
  Ta : Constant  Value=20
  Te : Constant  Value=-10
  Thermostat : Subsystem
  Watts : Constant  Value=Fridge_W
  Out1 : Outport  VectorParamsAs1DForOutWhenUnconnected=off
  wires:
  T_I/1 -> Add/2
  Add/1 -> Thermostat/1(In1), Scope/1, Divide3/1
  Integrator/1 -> Add/1
  Gain/1 -> Integrator/1
  Rec1/1 -> Switch/1
  Product3/1 -> Switch1/1
  Off/1 -> Switch1/3
  Rec/1 -> Product/2, Switch/3
  Ri/1 -> Product1/1
  Thermostat/1(Out1) -> Switch/2, Out1/1
  Te/1 -> Divide1/1
  Product2/1 -> Divide3/2
  Divide/1 -> Product3/1
  Divide3/1 -> Subtract/3
  Constant/1 -> Divide/2
  Divide2/1 -> Subtract/2
  Divide1/1 -> Product3/2
  Cc/1 -> Product/1, Product1/2
  Watts/1 -> Divide/1
  Ta/1 -> Divide2/1
  Product1/1 -> Divide2/2, Product2/1
  Product/1 -> Divide1/2
  In1/1 -> Switch1/2
  Switch1/1 -> Subtract/1
  Switch/1 -> Product2/2
  Subtract/1 -> Gain/1

== system Microgrid_W/House 5 W1/Shower/D1 ==
  Add : Sum  Inputs=+++
  Clock : Clock
  Constant : Constant
  Constant1 : Constant  Value=0
  Gain : Gain  Gain=t
  Interval Test : simulink/Logic and Bit Operations/Interval Test  IntervalClosedRight=on  uplimit=Shower_On_a+Shower_L_a  IntervalClosedLeft=on  lowlimit=Shower_On_a  OutDataTypeStr=boolean
  Interval Test1 : simulink/Logic and Bit Operations/Interval Test  IntervalClosedRight=on  uplimit=Shower_On_b+Shower_L_b  IntervalClosedLeft=on  lowlimit=Shower_On_b  OutDataTypeStr=boolean
  Interval Test2 : simulink/Logic and Bit Operations/Interval Test  IntervalClosedRight=on  uplimit=Shower_On_c+Shower_L_c  IntervalClosedLeft=on  lowlimit=Shower_On_c  OutDataTypeStr=boolean
  Switch : Switch  Criteria=u2 > Threshold  Threshold=0.5
  Switch1 : Switch  Criteria=u2 > Threshold  Threshold=0.5
  Switch2 : Switch  Criteria=u2 > Threshold  Threshold=0.5
  Out1 : Outport  VectorParamsAs1DForOutWhenUnconnected=off
  wires:
  Clock/1 -> Gain/1
  Add/1 -> Out1/1
  Interval Test2/1 -> Switch2/2
  Interval Test/1 -> Switch/2
  Interval Test1/1 -> Switch1/2
  Switch2/1 -> Add/3
  Switch1/1 -> Add/2
  Switch/1 -> Add/1
  Gain/1 -> Interval Test/1, Interval Test1/1, Interval Test2/1
  Constant/1 -> Switch/1, Switch2/1, Switch1/1
  Constant1/1 -> Switch/3, Switch1/3, Switch2/3

== system Microgrid_W/House 5 W1/Shower/D2 ==
  Add : Sum  Inputs=+++
  Clock : Clock
  Constant : Constant
  Constant1 : Constant  Value=0
  Gain : Gain  Gain=t
  Interval Test : simulink/Logic and Bit Operations/Interval Test  IntervalClosedRight=on  uplimit=Shower_On_a+(Shower_L_a+86400)  IntervalClosedLeft=on  lowlimit=Shower_On_a+86400  OutDataTypeStr=boolean
  Interval Test1 : simulink/Logic and Bit Operations/Interval Test  IntervalClosedRight=on  uplimit=Shower_On_b+(Shower_L_b+86400)  IntervalClosedLeft=on  lowlimit=Shower_On_b+86400  OutDataTypeStr=boolean
  Interval Test2 : simulink/Logic and Bit Operations/Interval Test  IntervalClosedRight=on  uplimit=Shower_On_c+(Shower_L_c+86400)  IntervalClosedLeft=on  lowlimit=Shower_On_c+86400  OutDataTypeStr=boolean
  Switch : Switch  Criteria=u2 > Threshold  Threshold=0.5
  Switch1 : Switch  Criteria=u2 > Threshold  Threshold=0.5
  Switch2 : Switch  Criteria=u2 > Threshold  Threshold=0.5
  Out1 : Outport  VectorParamsAs1DForOutWhenUnconnected=off
  wires:
  Clock/1 -> Gain/1
  Constant1/1 -> Switch2/3, Switch1/3, Switch/3
  Constant/1 -> Switch1/1, Switch2/1, Switch/1
  Gain/1 -> Interval Test2/1, Interval Test1/1, Interval Test/1
  Switch/1 -> Add/1
  Switch1/1 -> Add/2
  Switch2/1 -> Add/3
  Interval Test1/1 -> Switch1/2
  Interval Test/1 -> Switch/2
  Interval Test2/1 -> Switch2/2
  Add/1 -> Out1/1

== system Microgrid_W/House 5 W1/Shower/D3 ==
  Add : Sum  Inputs=+++
  Clock : Clock
  Constant : Constant
  Constant1 : Constant  Value=0
  Gain : Gain  Gain=t
  Interval Test : simulink/Logic and Bit Operations/Interval Test  IntervalClosedRight=on  uplimit=Shower_On_a+(Shower_L_a+86400*2)  IntervalClosedLeft=on  lowlimit=Shower_On_a+86400*2  OutDataTypeStr=boolean
  Interval Test1 : simulink/Logic and Bit Operations/Interval Test  IntervalClosedRight=on  uplimit=Shower_On_b+(Shower_L_b+86400*2)  IntervalClosedLeft=on  lowlimit=Shower_On_b+86400*2  OutDataTypeStr=boolean
  Interval Test2 : simulink/Logic and Bit Operations/Interval Test  IntervalClosedRight=on  uplimit=Shower_On_c+(Shower_L_c+86400*2)  IntervalClosedLeft=on  lowlimit=Shower_On_c+86400*2  OutDataTypeStr=boolean
  Switch : Switch  Criteria=u2 > Threshold  Threshold=0.5
  Switch1 : Switch  Criteria=u2 > Threshold  Threshold=0.5
  Switch2 : Switch  Criteria=u2 > Threshold  Threshold=0.5
  Out1 : Outport  VectorParamsAs1DForOutWhenUnconnected=off
  wires:
  Clock/1 -> Gain/1
  Add/1 -> Out1/1
  Interval Test2/1 -> Switch2/2
  Interval Test/1 -> Switch/2
  Interval Test1/1 -> Switch1/2
  Switch2/1 -> Add/3
  Switch1/1 -> Add/2
  Switch/1 -> Add/1
  Gain/1 -> Interval Test/1, Interval Test1/1, Interval Test2/1
  Constant/1 -> Switch/1, Switch2/1, Switch1/1
  Constant1/1 -> Switch/3, Switch1/3, Switch2/3

== system Microgrid_W/House 5 W1/Shower/D4 ==
  Add : Sum  Inputs=+++
  Clock : Clock
  Constant : Constant
  Constant1 : Constant  Value=0
  Gain : Gain  Gain=t
  Interval Test : simulink/Logic and Bit Operations/Interval Test  IntervalClosedRight=on  uplimit=Shower_On_a+Shower_L_a+86400*3  IntervalClosedLeft=on  lowlimit=Shower_On_a+86400*3  OutDataTypeStr=boolean
  Interval Test1 : simulink/Logic and Bit Operations/Interval Test  IntervalClosedRight=on  uplimit=Shower_On_b+Shower_L_b+86400*3  IntervalClosedLeft=on  lowlimit=Shower_On_b+86400*3  OutDataTypeStr=boolean
  Interval Test2 : simulink/Logic and Bit Operations/Interval Test  IntervalClosedRight=on  uplimit=Shower_On_c+Shower_L_c+86400*3  IntervalClosedLeft=on  lowlimit=Shower_On_c+86400*3  OutDataTypeStr=boolean
  Switch : Switch  Criteria=u2 > Threshold  Threshold=0.5
  Switch1 : Switch  Criteria=u2 > Threshold  Threshold=0.5
  Switch2 : Switch  Criteria=u2 > Threshold  Threshold=0.5
  Out1 : Outport  VectorParamsAs1DForOutWhenUnconnected=off
  wires:
  Clock/1 -> Gain/1
  Constant1/1 -> Switch2/3, Switch1/3, Switch/3
  Constant/1 -> Switch1/1, Switch2/1, Switch/1
  Gain/1 -> Interval Test2/1, Interval Test1/1, Interval Test/1
  Switch/1 -> Add/1
  Switch1/1 -> Add/2
  Switch2/1 -> Add/3
  Interval Test1/1 -> Switch1/2
  Interval Test/1 -> Switch/2
  Interval Test2/1 -> Switch2/2
  Add/1 -> Out1/1

== system Microgrid_W/House 5 W1/Shower/D5 ==
  Add : Sum  Inputs=+++
  Clock : Clock
  Constant : Constant
  Constant1 : Constant  Value=0
  Gain : Gain  Gain=t
  Interval Test : simulink/Logic and Bit Operations/Interval Test  IntervalClosedRight=on  uplimit=Shower_On_a+Shower_L_a+86400*4  IntervalClosedLeft=on  lowlimit=Shower_On_a+86400*4  OutDataTypeStr=boolean
  Interval Test1 : simulink/Logic and Bit Operations/Interval Test  IntervalClosedRight=on  uplimit=Shower_On_b+Shower_L_b+86400*4  IntervalClosedLeft=on  lowlimit=Shower_On_b+86400*4  OutDataTypeStr=boolean
  Interval Test2 : simulink/Logic and Bit Operations/Interval Test  IntervalClosedRight=on  uplimit=Shower_On_c+Shower_L_c+86400*4  IntervalClosedLeft=on  lowlimit=Shower_On_c+86400*4  OutDataTypeStr=boolean
  Switch : Switch  Criteria=u2 > Threshold  Threshold=0.5
  Switch1 : Switch  Criteria=u2 > Threshold  Threshold=0.5
  Switch2 : Switch  Criteria=u2 > Threshold  Threshold=0.5
  Out1 : Outport  VectorParamsAs1DForOutWhenUnconnected=off
  wires:
  Clock/1 -> Gain/1
  Add/1 -> Out1/1
  Interval Test2/1 -> Switch2/2
  Interval Test/1 -> Switch/2
  Interval Test1/1 -> Switch1/2
  Switch2/1 -> Add/3
  Switch1/1 -> Add/2
  Switch/1 -> Add/1
  Gain/1 -> Interval Test/1, Interval Test1/1, Interval Test2/1
  Constant/1 -> Switch/1, Switch2/1, Switch1/1
  Constant1/1 -> Switch/3, Switch1/3, Switch2/3

== system Microgrid_W/House 5 W1/Shower/D6 ==
  Add : Sum  Inputs=+++
  Clock : Clock
  Constant : Constant
  Constant1 : Constant  Value=0
  Gain : Gain  Gain=t
  Interval Test : simulink/Logic and Bit Operations/Interval Test  IntervalClosedRight=on  uplimit=Shower_On_a+Shower_L_a+86400*5  IntervalClosedLeft=on  lowlimit=Shower_On_a+86400*5  OutDataTypeStr=boolean
  Interval Test1 : simulink/Logic and Bit Operations/Interval Test  IntervalClosedRight=on  uplimit=Shower_On_b+Shower_L_b+86400*5  IntervalClosedLeft=on  lowlimit=Shower_On_b+86400*5  OutDataTypeStr=boolean
  Interval Test2 : simulink/Logic and Bit Operations/Interval Test  IntervalClosedRight=on  uplimit=Shower_On_c+Shower_L_c+86400*5  IntervalClosedLeft=on  lowlimit=Shower_On_c+86400*5  OutDataTypeStr=boolean
  Switch : Switch  Criteria=u2 > Threshold  Threshold=0.5
  Switch1 : Switch  Criteria=u2 > Threshold  Threshold=0.5
  Switch2 : Switch  Criteria=u2 > Threshold  Threshold=0.5
  Out1 : Outport  VectorParamsAs1DForOutWhenUnconnected=off
  wires:
  Clock/1 -> Gain/1
  Constant1/1 -> Switch2/3, Switch1/3, Switch/3
  Constant/1 -> Switch1/1, Switch2/1, Switch/1
  Gain/1 -> Interval Test2/1, Interval Test1/1, Interval Test/1
  Switch/1 -> Add/1
  Switch1/1 -> Add/2
  Switch2/1 -> Add/3
  Interval Test1/1 -> Switch1/2
  Interval Test/1 -> Switch/2
  Interval Test2/1 -> Switch2/2
  Add/1 -> Out1/1

== system Microgrid_W/House 5 W1/Shower/D7 ==
  Add : Sum  Inputs=+++
  Clock : Clock
  Constant : Constant
  Constant1 : Constant  Value=0
  Gain : Gain  Gain=t
  Interval Test : simulink/Logic and Bit Operations/Interval Test  IntervalClosedRight=on  uplimit=Shower_On_a+Shower_L_a+86400*6  IntervalClosedLeft=on  lowlimit=Shower_On_a+86400*6  OutDataTypeStr=boolean
  Interval Test1 : simulink/Logic and Bit Operations/Interval Test  IntervalClosedRight=on  uplimit=Shower_On_b+Shower_L_b+86400*6  IntervalClosedLeft=on  lowlimit=Shower_On_b+86400*6  OutDataTypeStr=boolean
  Interval Test2 : simulink/Logic and Bit Operations/Interval Test  IntervalClosedRight=on  uplimit=Shower_On_c+Shower_L_c+86400*6  IntervalClosedLeft=on  lowlimit=Shower_On_c+86400*6  OutDataTypeStr=boolean
  Switch : Switch  Criteria=u2 > Threshold  Threshold=0.5
  Switch1 : Switch  Criteria=u2 > Threshold  Threshold=0.5
  Switch2 : Switch  Criteria=u2 > Threshold  Threshold=0.5
  Out1 : Outport  VectorParamsAs1DForOutWhenUnconnected=off
  wires:
  Clock/1 -> Gain/1
  Add/1 -> Out1/1
  Interval Test2/1 -> Switch2/2
  Interval Test/1 -> Switch/2
  Interval Test1/1 -> Switch1/2
  Switch2/1 -> Add/3
  Switch1/1 -> Add/2
  Switch/1 -> Add/1
  Gain/1 -> Interval Test/1, Interval Test1/1, Interval Test2/1
  Constant/1 -> Switch/1, Switch2/1, Switch1/1
  Constant1/1 -> Switch/3, Switch1/3, Switch2/3
